simulink model "CP27E_TC"  (R2026a)
settings: Solver=ode23t  StopTime=10  MaxStep=0.001
undefined symbols (not defined in the file or in its folder): I0, X0
settings Model: Creator=jacks  LastModifiedBy=jacks

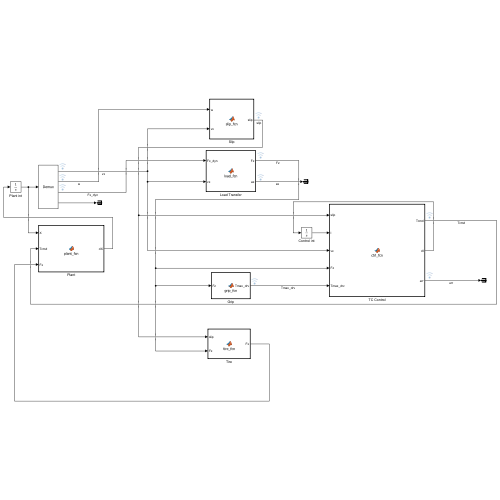
[thumbnail: Simulink's stored preview of the top-level diagram]
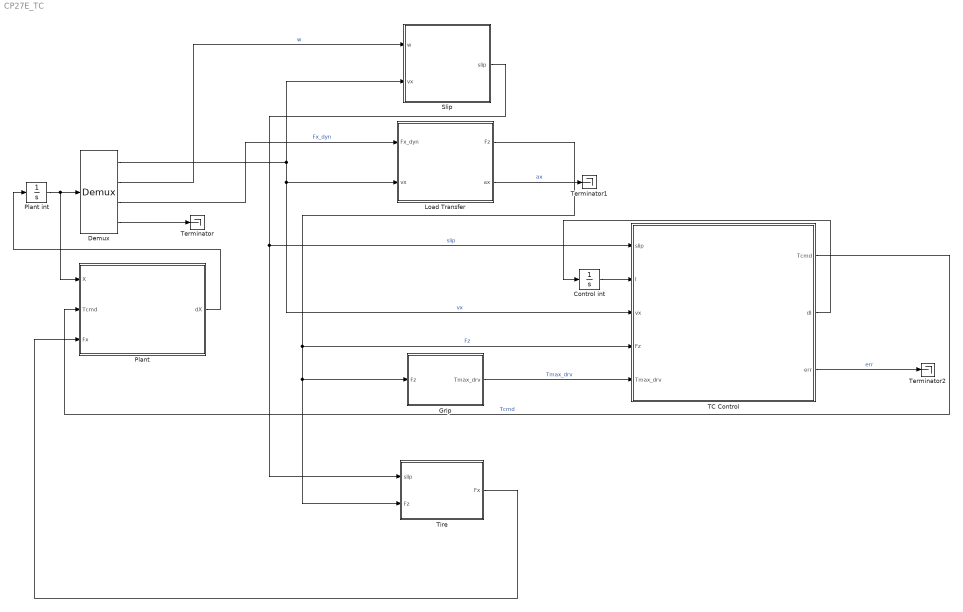
== system CP27E_TC ==
  Control int : Integrator  InitialCondition=I0
  Demux : Demux  Outputs=[1 4 4 4]
      settings: DisplayOption=none
  Grip : MATLAB Function  TreatAsAtomicUnit=on
  Load Transfer : MATLAB Function  TreatAsAtomicUnit=on
  Plant : MATLAB Function  TreatAsAtomicUnit=on
  Plant int : Integrator  InitialCondition=X0
  Slip : MATLAB Function  TreatAsAtomicUnit=on
  TC Control : MATLAB Function  TreatAsAtomicUnit=on
  Terminator : Terminator
  Terminator1 : Terminator
  Terminator2 : Terminator
  Tire : MATLAB Function  TreatAsAtomicUnit=on
  wires:
  Plant int/1 -> Plant/1(X), Demux/1
  Demux/1 -> TC Control/3(vx), Load Transfer/2(vx), Slip/2(vx)  "vx"
  Demux/2 -> Slip/1(w)  "w"
  Demux/3 -> Load Transfer/1(Fx_dyn)  "Fx_dyn"
  Demux/4 -> Terminator/1
  Slip/1(slip) -> Tire/1(slip), TC Control/1(slip)  "slip"
  Load Transfer/1(Fz) -> Tire/2(Fz), Grip/1(Fz), TC Control/4(Fz)  "Fz"
  Tire/1(Fx) -> Plant/3(Fx)
  Grip/1(Tmax_drv) -> TC Control/5(Tmax_drv)  "Tmax_drv"
  Control int/1 -> TC Control/2(I)
  TC Control/1(Tcmd) -> Plant/2(Tcmd)  "Tcmd"
  TC Control/2(dI) -> Control int/1
  Plant/1(dX) -> Plant int/1
  Load Transfer/2(ax) -> Terminator1/1  "ax"
  TC Control/3(err) -> Terminator2/1  "err"

== matlab function CP27E_TC/Slip ==
  data: w input; slip output; vx input
function slip = slip_fcn(w, vx)
  coder.extrinsic('evalin','slip_estimator');
  P = evalin('base','P');
  slip = zeros(1,4);
  slip = slip_estimator(w, vx, P);
end

== matlab function CP27E_TC/Load Transfer ==
  data: Fx_dyn input; Fz output; vx input; ax output
function [Fz, ax] = load_fcn(Fx_dyn, vx)
  coder.extrinsic('evalin','load_transfer');
  P = evalin('base','P');
  Fz = zeros(1,4); ax = 0;
  [Fz, ax] = load_transfer(Fx_dyn, vx, P);
end

== matlab function CP27E_TC/Tire ==
  data: slip input; Fx output; Fz input
function Fx = tire_fcn(slip, Fz)
  coder.extrinsic('evalin','tire_long');
  P = evalin('base','P');
  Fx = zeros(1,4);
  Fx = tire_long(slip, Fz, P);
end

== matlab function CP27E_TC/Grip ==
  data: Fz input; Tmax_drv output
function Tmax_drv = grip_fcn(Fz)
  coder.extrinsic('evalin','grip_estimator');
  P = evalin('base','P');
  Tmax_drv = zeros(1,4);
  Tmax_drv = grip_estimator(Fz, P);
end

== matlab function CP27E_TC/TC Control ==
  data: slip input; Tcmd output; I input; vx input; Fz input; Tmax_drv input; dI output; err output
function [Tcmd, dI, err] = ctrl_fcn(slip, I, vx, Fz, Tmax_drv)
  coder.extrinsic('evalin','tc_control');
  P = evalin('base','P');
  Tcmd=zeros(1,4); dI=zeros(1,4); err=zeros(1,4);
  [Tcmd, dI, err] = tc_control(slip, I, vx, Fz, Tmax_drv, P);
end

== matlab function CP27E_TC/Plant ==
  data: X input; dX output; Tcmd input; Fx input
function dX = plant_fcn(X, Tcmd, Fx)
  coder.extrinsic('evalin','plant_long');
  P = evalin('base','P');
  dX = zeros(13,1);
  dX = plant_long(X, Tcmd, Fx, P);
end
